simulink model "enable_hold"  (R2018a)
settings: Solver=FixedStepAuto  StartTime=0.0  StopTime=20  FixedStep=0.01  RelTol=1e-3
settings Model: EnablePacing=on  Creator=U500304  LastModifiedBy=U500304
settings SolverCC: ZeroCrossAlgorithm=Adaptive
settings DataIOCC: SaveOutput=off  SaveTime=off
settings DebuggingCC: MaxConsecutiveZCsMsg=none

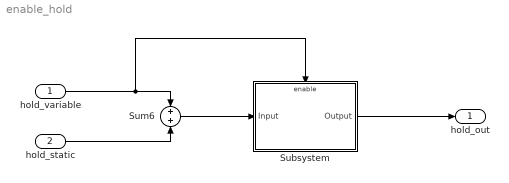
== system enable_hold ==
  hold_variable : Inport  OutDataTypeStr=double  PortDimensions=1  SampleTime=0
  hold_static : Inport  Port=2  OutDataTypeStr=double  PortDimensions=1
  Subsystem : Subsystem
  Sum6 : Sum
  hold_out : Outport  OutDataTypeStr=double  PortDimensions=1  SampleTime=0
  wires:
  Sum6/1 -> Subsystem/1(Input)
  Subsystem/1(Output) -> hold_out/1
  hold_static/1 -> Sum6/2
  hold_variable/1 -> Subsystem/Enable, Sum6/1

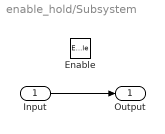
== system enable_hold/Subsystem ==
  Input : Inport
  Enable : EnablePort
  Output : Outport
  wires:
  Input/1 -> Output/1
